simulink library "lib_controller"  (Simulink 7.4)
settings: Solver=ode45  StartTime=0.0  StopTime=10.0  RelTol=1e-3
settings Model: Creator=chkajon  LastModifiedBy=chkajon

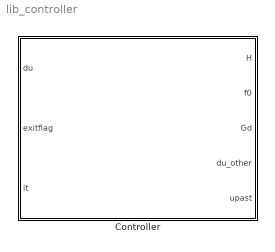
== system lib_controller ==
  Controller : Subsystem

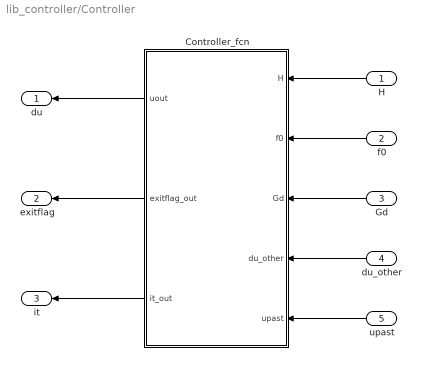
== system lib_controller/Controller ==
  H : Inport  OutDataType=fixdt(1, 16)  OutScaling=2^0
  f0 : Inport  Port=2  OutDataType=fixdt(1, 16)  OutScaling=2^0
  Gd : Inport  Port=3  OutDataType=fixdt(1, 16)  OutScaling=2^0
  du_other : Inport  Port=4  OutDataType=fixdt(1, 16)  OutScaling=2^0
  upast : Inport  Port=5  OutDataType=fixdt(1, 16)  OutScaling=2^0
  Controller_fcn : Stateflow chart  TreatAsAtomicUnit=on
  du : Outport  OutDataType=fixdt(1, 16)  OutScaling=2^0
  exitflag : Outport  Port=2  OutDataType=fixdt(1, 16)  OutScaling=2^0
  it : Outport  Port=3  OutDataType=fixdt(1, 16)  OutScaling=2^0
  wires:
  H/1 -> Controller_fcn/1(H)
  Gd/1 -> Controller_fcn/3(Gd)
  f0/1 -> Controller_fcn/2(f0)
  du_other/1 -> Controller_fcn/4(du_other)
  upast/1 -> Controller_fcn/5(upast)
  Controller_fcn/1(uout) -> du/1
  Controller_fcn/2(exitflag_out) -> exitflag/1
  Controller_fcn/3(it_out) -> it/1

== matlab function Controller/Controller_fcn ==
  data: H input double; f0 input double; Gd input double; du_other input double; upast input double; uout output double; exitflag_out output double; it_out output double
function [uout,exitflag_out,it_out]  = fcn(H, f0, Gd, du_other, upast)
%#eml
% persistent C_new M LB UB Ga Gb Gc H Ain b A B upast xinit
persistent LB UB Ain b
eml.extrinsic('disp');
eml.extrinsic('toc');
eml.extrinsic('tic');
eml.extrinsic('num2str');
eml.extrinsic('keyboard');

[~,~,usize,~,m] = const_mpc();


if isempty(LB)
    tic
    [~,~,UB,LB,b,Ain] = get_constant_matrices();
    time = toc;
    disp(['Preparation time: ' num2str(time)]);
end

% Get reference and input vector
Upast = zeros(m*usize,1);
for i=1:m
    Upast(1+(i-1)*usize:i*usize,1) = upast;
end

% Update bounds
LBa = LB - Upast;
UBa = UB - Upast;

% Update linear term to add effect of other compressor
f = f0 + du_other'*Gd;

% Solve QP
lbA = -inf(size(Ain,1),1);
[usol,~,exitflag,it] = call_qpoases_m(H,f,Ain,LBa,UBa,lbA,b);
exitflag_out = exitflag(1,1);
it_out = it(1,1);

if exitflag_out~=0
    exitflag_out
    usol = zeros(m*usize,1);
end

% Output
uout = zeros(m*usize,1);
for i=1:m*usize
    uout(i) = usol(i);
end
